simulink model "anders_spaceship_kin_temp"  (R2024b)
settings: Solver=ode45  StartTime=0.0  StopTime=20  RelTol=1e-3  EnableMultiTasking=on
libraries: sharedtransform x2, vrlib x2, simulink_extras x1
Description:
  | Plane Take-Off with HUD Text
  | 
  | This model is a variant of the vrtkoff example that shows also how to display
  | signal values as text in the virtual scene and a simple Head-Up Display (HUD).
  | 
  | The text is sent to the virtual world as Simulink(R) string signal, composed from the numeric
  | input values using the format string (see sprintf for more information) and sent
  | to the 'string' field of the corresponding Text node in the world. Individual lines of
  | the MFString field are separated by the newline character in the format string.
  | 
  | The HUD behavior (maintaining constant relative position between the user and the
  | Text node) is achieved by defining a ProximitySensor that senses user position and
  | orientation as it navigates through the scene and routing this information to the translation
  | and rotation of HUD object - in this case a VRML Transform that contains the Text node.
settings Model: Creator=The MathWorks, Inc.  LastModifiedBy=ander
settings SolverCC: ZeroCrossAlgorithm=Adaptive  AlgebraicLoopSolver=TrustRegion
settings DataIOCC: LimitDataPoints=on  SaveFormat=Array  SaveOutput=off  SaveTime=off  ReturnWorkspaceOutputs=off  SignalLoggingName=logsOut
settings OptimizationCC: BlockReduction=off  BooleanDataType=off  ExpressionDepthLimit=2147483647  InitFltsAndDblsToZero=on  LifeSpan=inf
settings DebuggingCC: UnderspecifiedInitializationDetection=Classic  MergeDetectMultiDrivingBlocksExec=none  CheckExecutionContextPreStartOutputMsg=on  SignalResolutionControl=TryResolveAllWithWarning  IgnoredZcDiagnostic=none  MultiTaskDSMMsg=warning  MultiTaskCondExecSysMsg=none  FcnCallInpInsideContextMsg=warning  UnconnectedInputMsg=warning  UnconnectedOutputMsg=warning  UnconnectedLineMsg=warning  StateNameClashWarn=warning  SymbolicDimsDataTypeCodeGenerationDiagnostic=none  SFUnexpectedBacktrackingDiag=warning  SFNoUnconditionalDefaultTransitionDiag=warning  SFExecutionAtInitializationDiag=none  ArithmeticOperatorsInVariantConditions=warning
settings HardwareCC: ProdBitPerPointer=32  ProdBitPerSizeT=32  ProdBitPerPtrDiffT=32  ProdLargestAtomicFloat=None  ProdIntDivRoundTo=Undefined  ProdEndianess=Unspecified  ProdWordSize=32  ProdHWDeviceType=32-bit Generic  TargetUnknown=on
settings ModelReferenceCC: UpdateModelReferenceTargets=IfOutOfDate  EnableRefExpFcnMdlSchedulingChecks=on  PropagateSignalLabelsOutOfModel=off
settings SFSimCC: SimUseLocalCustomCode=off  CustomCodeUndefinedFunction=UseInterfaceOnly
settings RTWCC: RTWUseLocalCustomCode=off  GPUComputeCapability=3.5  DLArmComputeVersion=19.05
settings CodeAppCC: StateflowObjectComments=on
settings GRTTargetCC: TargetFcnLib=ansi_tfl_tmw.mat  TargetLangStandard=C89/C90 (ANSI)  CombineOutputUpdateFcns=off  GRTInterface=on
settings ConfigComp: CovMetricSettings=d  CovSaveCumulativeToWorkspaceVar=on  CovSaveSingleToWorkspaceVar=on  CovExternalEMLEnable=off  CovSFcnEnable=off

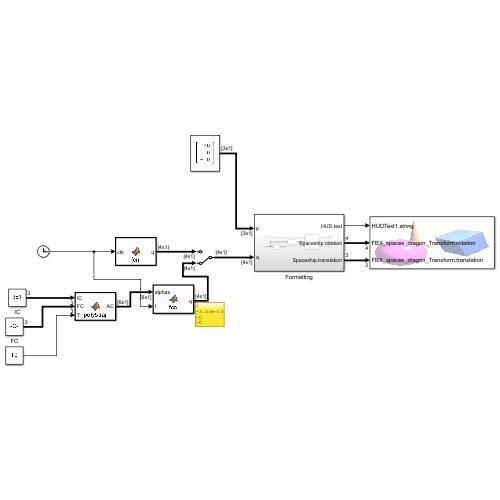
[thumbnail: Simulink's stored preview of the top-level diagram]
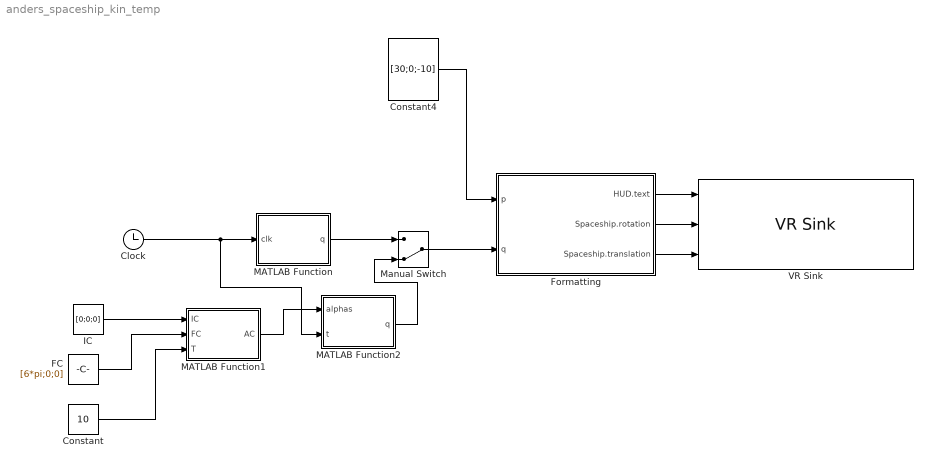
== system anders_spaceship_kin_temp ==
  Clock : Clock
  Constant : Constant  Value=10
  Constant4 : Constant  Value=[30;0;-10]  VectorParams1D=off
  FC : Constant  Value=[6*pi;0;0]
  Formatting : Subsystem
  IC : Constant  Value=[0;0;0]
  MATLAB Function : MATLAB Function  TreatAsAtomicUnit=on
  MATLAB Function1 : MATLAB Function  TreatAsAtomicUnit=on
  MATLAB Function2 : MATLAB Function  TreatAsAtomicUnit=on
  Manual Switch : ManualSwitch  CurrentSetting=0
  VR Sink : vrlib/VR Sink  InstantiateOnLoad=on  SampleTime=0.1  ViewEnable=on  RemoteChange=off  RemoteView=off  FieldsWritten=HUDText1.string.1.-1.1.char#FBX_spacex_dragon_Transform.rotation.4.1.1.double#FBX_spacex_dragon_Transform.translation.3.1.1.double  WorldFileName=spaceship_VR.x3d  WorldDescription=VR Spaceship Dragon  AutoView=off  VideoDimensions=[]  AllowVariableSize=off
  wires:
  Formatting/1(HUD.text) -> VR Sink/1
  Formatting/2(Spaceship.rotation) -> VR Sink/2
  Formatting/3(Spaceship.translation) -> VR Sink/3
  Constant4/1 -> Formatting/1(p)
  Clock/1 -> MATLAB Function2/2(t), MATLAB Function/1(clk)
  MATLAB Function/1(q) -> Manual Switch/1
  Manual Switch/1 -> Formatting/2(q)
  IC/1 -> MATLAB Function1/1(IC)
  FC/1 -> MATLAB Function1/2(FC)
  Constant/1 -> MATLAB Function1/3(T)
  MATLAB Function1/1(AC) -> MATLAB Function2/1(alphas)
  MATLAB Function2/1(q) -> Manual Switch/2

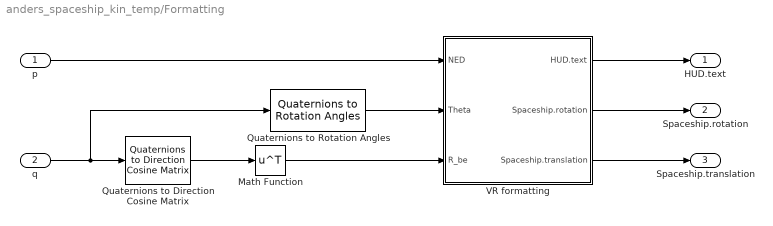
== system anders_spaceship_kin_temp/Formatting ==
  p : Inport
  q : Inport  Port=2
  Math Function : Math  Operator=transpose
  Quaternions to Direction Cosine Matrix : sharedtransform/Quaternions to  Direction Cosine Matrix  aMode=aMode
      settings: LibrarySourceBlock=|
      | aerolibtransform2/Quaternions to
      | Direction Cosine Matrix
  Quaternions to Rotation Angles : sharedtransform/Quaternions to Rotation Angles  rotationOrder=XYZ  aMode=aMode
  VR formatting : Subsystem
  HUD.text : Outport
  Spaceship.rotation : Outport  Port=2
  Spaceship.translation : Outport  Port=3
  wires:
  VR formatting/1(HUD.text) -> HUD.text/1
  VR formatting/2(Spaceship.rotation) -> Spaceship.rotation/1
  VR formatting/3(Spaceship.translation) -> Spaceship.translation/1
  p/1 -> VR formatting/1(NED)
  Math Function/1 -> VR formatting/3(R_be)
  Quaternions to Direction Cosine Matrix/1 -> Math Function/1
  q/1 -> Quaternions to Rotation Angles/1, Quaternions to Direction Cosine Matrix/1
  Quaternions to Rotation Angles/1 -> VR formatting/2(Theta)

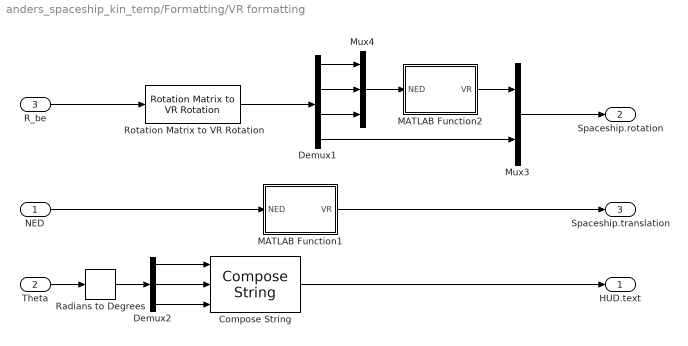
== system anders_spaceship_kin_temp/Formatting/VR formatting ==
  NED : Inport
  Theta : Inport  Port=2
  R_be : Inport  Port=3
  Compose String : ComposeString  Format="'Roll    : %7.2f deg\\nPitch   : %7.2f deg\\nYaw     : %7.2f deg'"
  Demux1 : Demux
  Demux2 : Demux  Outputs=3
  MATLAB Function1 : MATLAB Function  TreatAsAtomicUnit=on
  MATLAB Function2 : MATLAB Function  TreatAsAtomicUnit=on
  Mux3 : Mux  Inputs=2
  Mux4 : Mux  Inputs=3
  Radians to Degrees : simulink_extras/Transformations/Radians to Degrees
  Rotation Matrix to VR Rotation : vrlib/Utilities/Rotation Matrix to VR Rotation  maxzero=1e-12
  HUD.text : Outport
  Spaceship.rotation : Outport  Port=2
  Spaceship.translation : Outport  Port=3
  wires:
  Rotation Matrix to VR Rotation/1 -> Demux1/1
  Mux3/1 -> Spaceship.rotation/1
  MATLAB Function2/1(VR) -> Mux3/1
  Mux4/1 -> MATLAB Function2/1(NED)
  Demux1/3 -> Mux4/3
  Demux1/1 -> Mux4/1
  Demux1/2 -> Mux4/2
  Demux1/4 -> Mux3/2
  NED/1 -> MATLAB Function1/1(NED)
  MATLAB Function1/1(VR) -> Spaceship.translation/1
  Demux2/1 -> Compose String/1
  Demux2/2 -> Compose String/2
  Demux2/3 -> Compose String/3
  Compose String/1 -> HUD.text/1
  Theta/1 -> Radians to Degrees/1
  R_be/1 -> Rotation Matrix to VR Rotation/1
  Radians to Degrees/1 -> Demux2/1

== matlab function anders_spaceship_kin_temp/MATLAB Function1 ==
  data: IC input; AC output; FC input; T input
function AC = poly5traj(IC,FC,T)

%POLY5TRAJ Computes coefficients of polynomial for trajectory planning.
%   AC = POLY5TRAJ(IC,FC,T) finds the vector AC of the coefficients of a 
%   polynomial h(t) of degree 5 (h(t)=AC(1)+AC(2)*t+AC(3)*t^2+...+AC(6)*T^5), 
%   with initial conditions being specified in the vector IC=[h(0);h^(1)(0);h^(2)(0)], 
%   and final conditions at time t=T specified in the vector 
%   FC=[h(T);h^(1)(T);h^(2)(T)].

%   Jerome Jouffroy, January 2023

AC = zeros(6,1);

AC(1) = IC(1); % alpha 0
AC(2) = IC(2); % alpha 1
AC(3) = IC(3)/2; % alpha 2

Tmatrix = [ T^3      ,    T^4  , T^5        ;
            3*T^3    ,   4*T^4 ,  5*T^5     ;
            2*3*T^3  ,3*4*T^4  ,4*5*T^5   ];
        
AC(4:6,1) = inv(Tmatrix)*[ FC(1)-(AC(1)+AC(2)*T+AC(3)*T^2) ;
                            T*(FC(2)-(AC(2)+2*AC(3)*T));
                            T^2*(FC(3)-2*AC(3)) ];

== matlab function anders_spaceship_kin_temp/MATLAB Function ==
  data: q output; clk input
function q = fcn(clk)

n_rot = 3;
total_time = 10;

beta = clk*n_rot*(2*pi)/total_time;

ax =  [1;20;13];
k = ax/norm(ax);

eta = cos(beta/2);
epsilon = k*sin(beta/2);

q = [   eta;
        epsilon ];

== matlab function anders_spaceship_kin_temp/MATLAB Function2 ==
  data: alphas input; q output; t input
function q = fcn(alphas, t)

beta = alphas(1) + alphas(2)*t + alphas(3)*t^2 + alphas(4)*t^3 + alphas(5)*t^4 + alphas(6)*t^5;

k = [
        1;
        0;
        0
            ];

q = [
        cos(beta/2);
        k*sin(beta/2)
            ];

== matlab function anders_spaceship_kin_temp/Formatting/VR formatting/MATLAB Function1 ==
  data: NED input; VR output
function VR = NED2VR(NED)

x = NED(1); % north
y = NED(2); % east 
z = NED(3); % down

VR = [ -y ; -z ; x ];

== matlab function anders_spaceship_kin_temp/Formatting/VR formatting/MATLAB Function2 ==
  data: NED input; VR output
function VR = NED2VR(NED)

x = NED(1); % north
y = NED(2); % east 
z = NED(3); % down

VR = [ -y ; -z ; x ];
